simulink model "LADRC_SIMU_R1"  (R2018b)
settings: Solver=VariableStepAuto  StartTime=0.0  StopTime=10.0  RelTol=1e-3
settings Model: Creator=Whtest  LastModifiedBy=Risky Jr

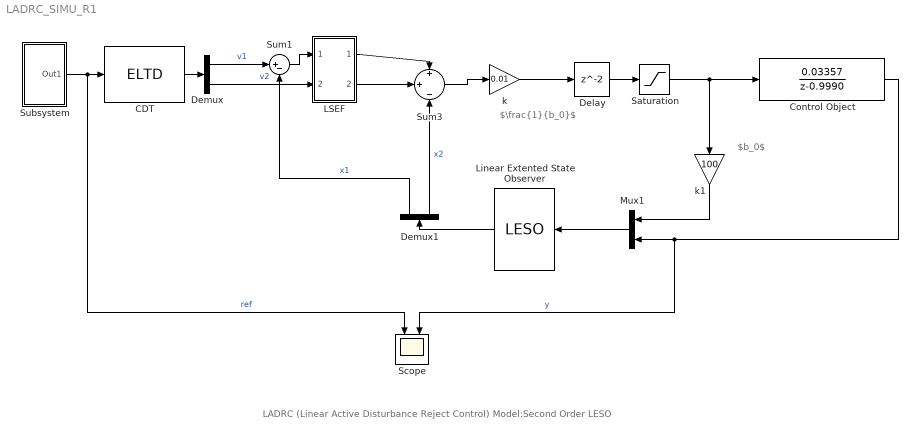
== system LADRC_SIMU_R1 ==
  note: LADRC (Linear Active Disturbance Reject Control)
      | Model:Second Order LESO
  note: $\frac{1}{b_0}$
  note: $b_0$
  CDT : S-Function  FunctionName=ELTD  Parameters=4,4.8,100  SFunctionDeploymentMode=off  EnableBusSupport=off
  Control Object : DiscreteTransferFcn  Numerator="[0    0.03357]"  Denominator="[ 1.0000   -0.9990]"  SampleTime=1e-3
  Delay : Delay
  Demux : Demux  Outputs=2
  Demux1 : Demux  Outputs=2
  LSEF : Subsystem
  Linear Extented State Observer : S-Function  FunctionName=LESO  Parameters=100  SFunctionDeploymentMode=off  EnableBusSupport=off
  Mux1 : Mux  Inputs=2
  Saturation : Saturate  UpperLimit=1e5  LowerLimit=-1e5
  Scope : Scope  NumInputPorts=2
  Subsystem : Subsystem
  Sum1 : Sum  Inputs=|+-
  Sum3 : Sum  Inputs=+|+|-
  k : Gain  Gain=0.01
  k1 : Gain  Gain=100
  wires:
  Control Object/1 -> Mux1/2, Scope/2  "y"
  CDT/1 -> Demux/1
  Demux/1 -> Sum1/1  "v1"
  Sum1/1 -> LSEF/1(In1)
  Mux1/1 -> Linear Extented State Observer/1
  k/1 -> Delay/1
  Demux/2 -> LSEF/2(In2)  "v2"
  Linear Extented State Observer/1 -> Demux1/1
  LSEF/1(Out1) -> Sum3/1
  LSEF/2(Out2) -> Sum3/2
  Sum3/1 -> k/1
  Demux1/2 -> Sum3/3  "x2"
  Saturation/1 -> k1/1, Control Object/1
  k1/1 -> Mux1/1
  Demux1/1 -> Sum1/2  "x1"
  Delay/1 -> Saturation/1
  Subsystem/1(Out1) -> Scope/1, CDT/1  "ref"

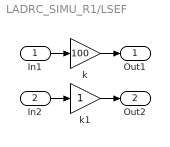
== system LADRC_SIMU_R1/LSEF ==
  In1 : Inport
  In2 : Inport  Port=2
  k : Gain  Gain=100
  k1 : Gain
  Out1 : Outport
  Out2 : Outport  Port=2
  wires:
  In1/1 -> k/1
  In2/1 -> k1/1
  k/1 -> Out1/1
  k1/1 -> Out2/1

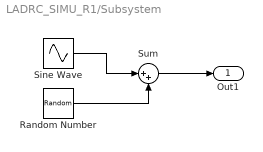
== system LADRC_SIMU_R1/Subsystem ==
  Random Number : RandomNumber  Variance=0.01  SampleTime=1e-3
  Sine Wave : Sin  Frequency=6.28  SampleTime=1e-3
  Sum : Sum  Inputs=|++
  Out1 : Outport
  wires:
  Sine Wave/1 -> Sum/1
  Random Number/1 -> Sum/2
  Sum/1 -> Out1/1
